simulink model "openloopHbridgedrive"  (R2016a)
settings: Solver=ode3  SolverMode=SingleTasking  StartTime=0.0  StopTime=inf  RelTol=1e-3
libraries: arduinolib x3, dspadpt3 x1
settings Model: SimulationMode=external  ExtModeTrigDuration=2  Creator=dell  LastModifiedBy=dell
settings DataIOCC: LimitDataPoints=on  SaveFormat=Array
settings OptimizationCC: OptimizeModelRefInitCode=on  LifeSpan=1  MaxStackSize=64
settings DebuggingCC: UnderspecifiedInitializationDetection=Classic  MergeDetectMultiDrivingBlocksExec=none  StateNameClashWarn=warning
settings HardwareCC: ProdBitPerInt=16  ProdBitPerPointer=16  ProdLargestAtomicFloat=None  ProdWordSize=8  ProdHWDeviceType=Atmel->AVR
settings ModelReferenceCC: PropagateSignalLabelsOutOfModel=off
settings RTWCC: SystemTargetFile=ert.tlc  HardwareBoard=Arduino Mega 2560  TemplateMakefile=ert_default_tmf  GenerateReport=on  RTWVerbose=off  Toolchain=Arduino AVR v1.6.1  BuildConfiguration=Faster Runs  IncludeHyperlinkInReport=on  LaunchReport=on  GenerateTraceInfo=on  GenerateTraceReport=on  GenerateTraceReportSl=on  GenerateTraceReportSf=on  GenerateTraceReportEml=on
settings CodeAppCC: ForceParamTrailComments=on  IgnoreCustomStorageClasses=off  OperatorAnnotations=on  SimulinkDataObjDesc=on  SFDataObjDesc=on  MATLABFcnDesc=on  MangleLength=10  InsertBlockDesc=on  MATLABSourceComments=on
settings ERTTargetCC: SupportContinuousTime=on  SupportVariableSizeSignals=on  ExtMode=on  ExtModeTransport=3  ExtModeMexFile=ext_serial_win32_comm_rtt  ExtModeMexArgs=0 5 115200
settings ConfigComp: CovModelRefEnable=Off

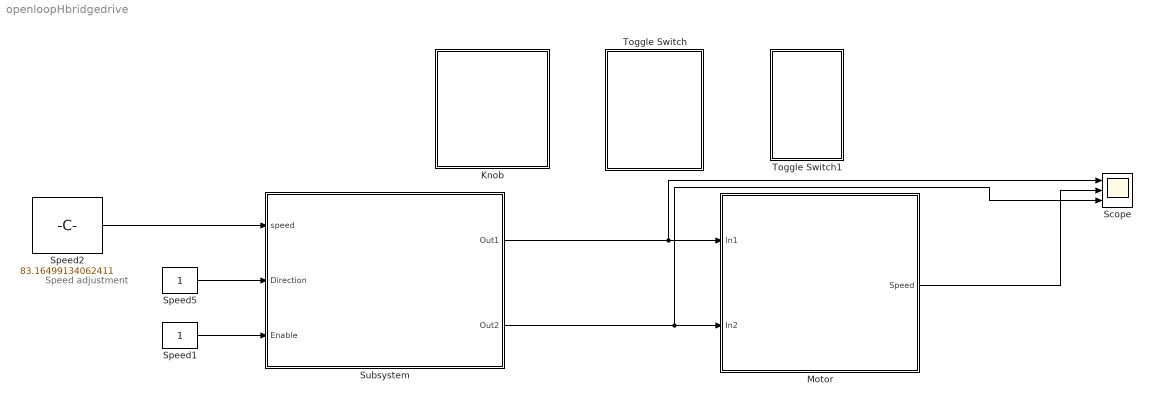
== system openloopHbridgedrive ==
  note: Speed adjustment
  Knob : Subsystem  DialogController=hmiCreateDDGDialog  IsWebBlock=on  mask(MWDashboardBlock){webBlockId=bad20c72-3a81-465b-aca1-27ab5a06c83c, webBlockType=continuousknob, ShowInLibBrowser=on, ShowInitialText=on, HMISrcModelName=openloopHbridgedrive}
      mask prompts: webBlockId "WebBlock Id"; webBlockType "WebBlock Type"; HMISrcModelName "Source Model"
      mask Help: helpview([docroot '/mapfiles/simulink.map'], 'hmi_knob')
      mask Display:
      | if strcmp(get_param(bdroot(gcb),'BlockDiagramType'), 'library')
      |     image([(matlabroot) '/toolbox/simulink/hmi/icons/ContinuousKnob.png']);
      | end
  Motor : Subsystem
  Scope : Scope  NumInputPorts=3
  Speed1 : Constant  OutMin=0  OutMax=100  OutDataTypeStr=single  SampleTime=0.001
  Speed2 : Constant  Value=83.16499134062411  OutMin=0  OutMax=100  OutDataTypeStr=single  SampleTime=0.001
  Speed5 : Constant  OutMin=0  OutMax=100  OutDataTypeStr=single  SampleTime=0.001
  Subsystem : Subsystem
  Toggle Switch : Subsystem  DialogController=hmiCreateDDGDialog  IsWebBlock=on  mask(MWDashboardBlock){webBlockId=f6c8166b-2cab-402f-842a-ce216d7d2c82, webBlockType=toggleswitch, ShowInLibBrowser=on, ShowInitialText=on, HMISrcModelName=openloopHbridgedrive}
      mask prompts: webBlockId "WebBlock Id"; webBlockType "WebBlock Type"; HMISrcModelName "Source Model"
      mask Help: helpview([docroot '/mapfiles/simulink.map'], 'hmi_toggle_switch')
      mask Display:
      | if strcmp(get_param(bdroot(gcb),'BlockDiagramType'), 'library')
      |     image([(matlabroot) '/toolbox/simulink/hmi/icons/ToggleSwitch.png']);
      | end
  Toggle Switch1 : Subsystem  DialogController=hmiCreateDDGDialog  IsWebBlock=on  mask(MWDashboardBlock){webBlockId=53eccea4-bc18-4898-a6d0-165afc14bbde, webBlockType=toggleswitch, ShowInLibBrowser=on, ShowInitialText=on, HMISrcModelName=openloopHbridgedrive}
      mask prompts: webBlockId "WebBlock Id"; webBlockType "WebBlock Type"; HMISrcModelName "Source Model"
      mask Help: helpview([docroot '/mapfiles/simulink.map'], 'hmi_toggle_switch')
      mask Display:
      | if strcmp(get_param(bdroot(gcb),'BlockDiagramType'), 'library')
      |     image([(matlabroot) '/toolbox/simulink/hmi/icons/ToggleSwitch.png']);
      | end
  wires:
  Speed5/1 -> Subsystem/2(Direction)
  Subsystem/1(Out1) -> Scope/1, Motor/1(In1)
  Subsystem/2(Out2) -> Scope/3, Motor/2(In2)
  Speed1/1 -> Subsystem/3(Enable)
  Speed2/1 -> Subsystem/1(speed)
  Motor/1(Speed) -> Scope/2

== system openloopHbridgedrive/Knob ==

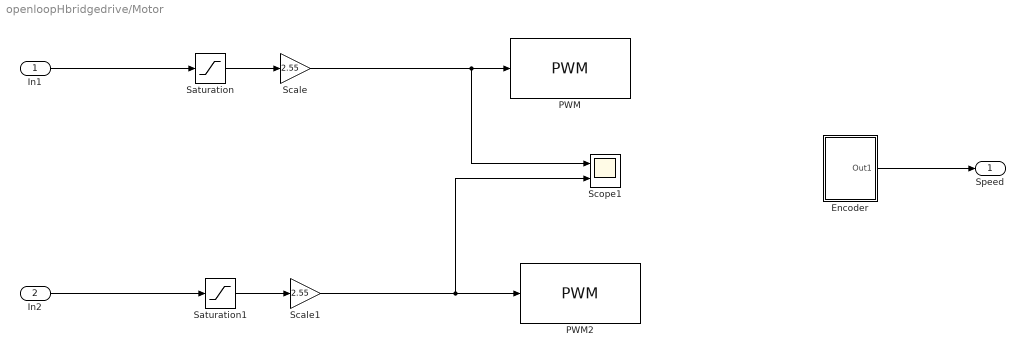
== system openloopHbridgedrive/Motor ==
  In1 : Inport
  In2 : Inport  Port=2
  "Encoder " : Subsystem
  PWM : arduinolib/PWM  pinNumber=5  blockPlatform=arduino
  PWM2 : arduinolib/PWM  pinNumber=4  blockPlatform=arduino
  Saturation : Saturate  UpperLimit=100  LowerLimit=0
      settings: AttributesFormatString=max = %<UpperLimit>\nmin = %<LowerLimit>
  Saturation1 : Saturate  UpperLimit=100  LowerLimit=0
      settings: AttributesFormatString=max = %<UpperLimit>\nmin = %<LowerLimit>
  Scale : Gain  Gain=2.55
  Scale1 : Gain  Gain=2.55
  Scope1 : Scope  NumInputPorts=2
  Speed : Outport
  wires:
  Saturation1/1 -> Scale1/1
  Scale1/1 -> Scope1/2, PWM2/1
  In1/1 -> Saturation/1
  In2/1 -> Saturation1/1
  Scale/1 -> Scope1/1, PWM/1
  Saturation/1 -> Scale/1
  "Encoder "/1(Out1) -> Speed/1

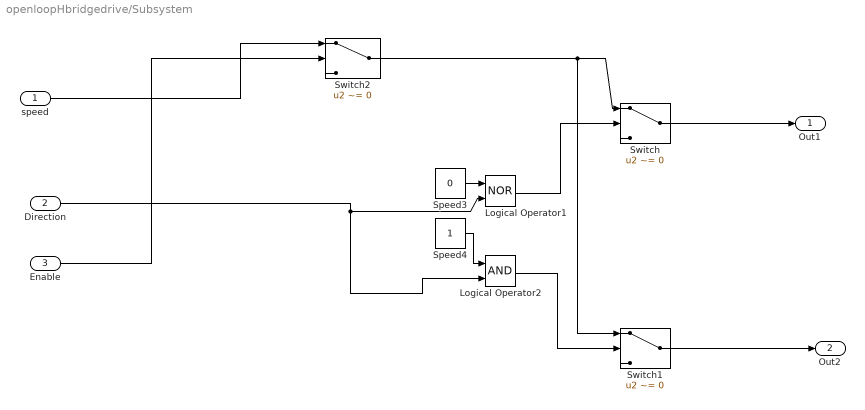
== system openloopHbridgedrive/Subsystem ==
  speed : Inport
  Direction : Inport  Port=2
  Enable : Inport  Port=3
  Logical Operator1 : Logic  Operator=NOR  AllPortsSameDT=off  OutDataTypeStr=boolean
  Logical Operator2 : Logic  AllPortsSameDT=off  OutDataTypeStr=boolean
  Speed3 : Constant  Value=0  OutMin=0  OutMax=100  OutDataTypeStr=single  SampleTime=0.001
  Speed4 : Constant  OutMin=0  OutMax=100  OutDataTypeStr=single  SampleTime=0.001
  Switch : Switch  Criteria=u2 ~= 0
  Switch1 : Switch  Criteria=u2 ~= 0
  Switch2 : Switch  Criteria=u2 ~= 0
  Out1 : Outport
  Out2 : Outport  Port=2
  wires:
  Logical Operator2/1 -> Switch1/2
  Speed4/1 -> Logical Operator2/1
  Direction/1 -> Logical Operator2/2, Logical Operator1/2
  Switch/1 -> Out1/1
  Switch1/1 -> Out2/1
  Logical Operator1/1 -> Switch/2
  speed/1 -> Switch2/1
  Speed3/1 -> Logical Operator1/1
  Enable/1 -> Switch2/2
  Switch2/1 -> Switch1/1, Switch/1

== system openloopHbridgedrive/Toggle Switch ==

== system openloopHbridgedrive/Toggle Switch1 ==

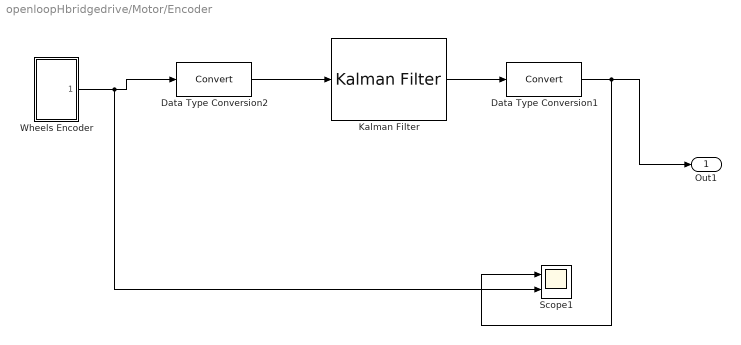
== system openloopHbridgedrive/Motor/Encoder  ==
  " Wheels Encoder" : Subsystem  AncestorBlock=closedloop/Right Wheels Encoder
  Data Type Conversion1 : DataTypeConversion
  Data Type Conversion2 : DataTypeConversion
  Kalman Filter : dspadpt3/Kalman Filter  num_targets=1  sourceEnable=Always  isReset=on  X=zeros([1])  P=10*eye(1)  A=[1]  sourceMeasure=Specify via Dialog  H=[1]  Q=0.0005*eye(1)  R=eye(1)  isOutputEstMeasure=on  isOutputEstState=off  isOutputEstError=off  isOutputPrdMeasure=off  isOutputPrdState=off  isOutputPrdError=off
  Scope1 : Scope  NumInputPorts=2
  Out1 : Outport
  wires:
  " Wheels Encoder"/1(Encoder) -> Scope1/2, Data Type Conversion2/1
  Data Type Conversion2/1 -> Kalman Filter/1
  Kalman Filter/1 -> Data Type Conversion1/1
  Data Type Conversion1/1 -> Scope1/1, Out1/1

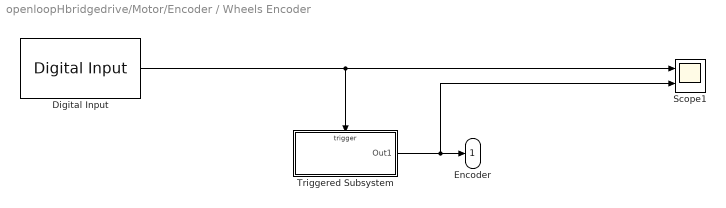
== system openloopHbridgedrive/Motor/Encoder / Wheels Encoder ==
  Digital Input : arduinolib/Digital Input  pinNumber=2  sampleTime=0.001  blockPlatform=arduino
  Scope1 : Scope  NumInputPorts=2
  Triggered Subsystem : Subsystem  TreatAsAtomicUnit=on
  Encoder : Outport
  wires:
  Digital Input/1 -> Triggered Subsystem/Trigger, Scope1/1
  Triggered Subsystem/1(Out1) -> Scope1/2, Encoder/1

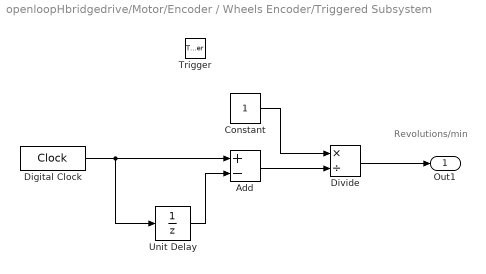
== system openloopHbridgedrive/Motor/Encoder / Wheels Encoder/Triggered Subsystem ==
  note: Revolutions/min
  Trigger : TriggerPort  VariantControl=Variant
  Add : Sum  Inputs=+-
  Constant : Constant
  Digital Clock : DigitalClock  SampleTime=-1
  Divide : Product  Inputs=*/  OutDataTypeStr=int32
  Unit Delay : UnitDelay  SampleTime=-1
  Out1 : Outport
  wires:
  Constant/1 -> Divide/1
  Divide/1 -> Out1/1
  Add/1 -> Divide/2
  Unit Delay/1 -> Add/2
  Digital Clock/1 -> Unit Delay/1, Add/1
